simulink subsystem "Pesudo_Transport"  (R2024a)
settings: Solver=VariableStepAuto  StartTime=0.0  StopTime=10.0  RelTol=1e-3
undefined symbols (not defined in the file): C0, coreFuelVolume, lam, N1, N2, outCoreFuelVolume, tau_l
settings Model: Creator=silen  LastModifiedBy=silen

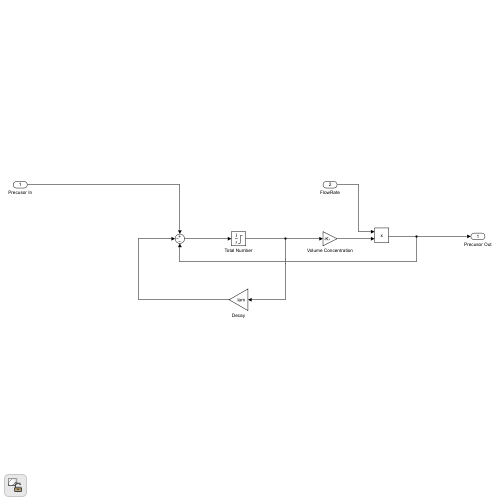
[thumbnail: Simulink's stored preview of the top-level diagram]
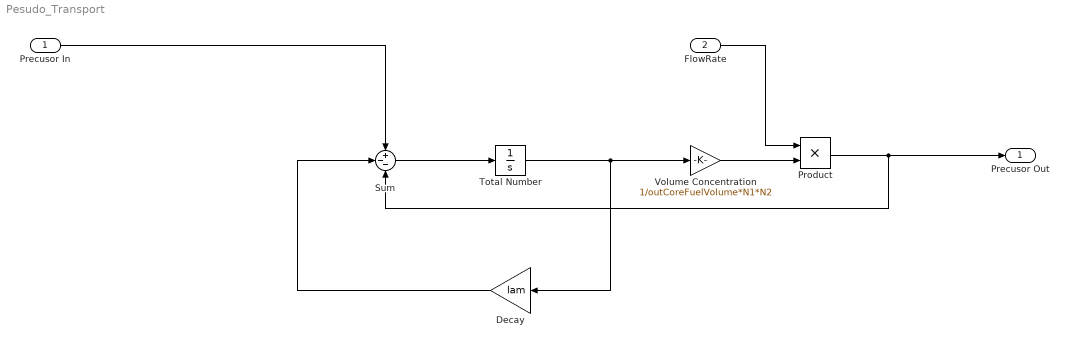
== system Pesudo_Transport ==
  Precusor In : Inport
  FlowRate : Inport  Port=2
  Decay : Gain  Gain=lam
  Product : Product
  Sum : Sum  Inputs=+--
  Total Number : Integrator  InitialCondition=C0.*exp(-lam*0.1*tau_l)/coreFuelVolume*outCoreFuelVolume/N1/N2  LimitOutput=on  LowerSaturationLimit=[0,0,0,0,0,0]
  Volume Concentration : Gain  Gain=1/outCoreFuelVolume*N1*N2
  Precusor Out : Outport
  wires:
  Total Number/1 -> Volume Concentration/1, Decay/1
  Sum/1 -> Total Number/1
  Precusor In/1 -> Sum/1
  Decay/1 -> Sum/2
  Product/1 -> Precusor Out/1, Sum/3
  FlowRate/1 -> Product/1
  Volume Concentration/1 -> Product/2
